simulink model "sistemaConControladorPID_R2022a"  (R2022a)
settings: Solver=VariableStepAuto  StartTime=0.0  StopTime=Ts  RelTol=1e-3
libraries: dspsrcs4 x1, slpidlib x1, cstblocks x1
settings Model: Creator=chris  LastModifiedBy=chris
settings ModelReferenceCC: EnableRefExpFcnMdlSchedulingChecks=off
settings RTWCC: Description=Generic Real-Time Target

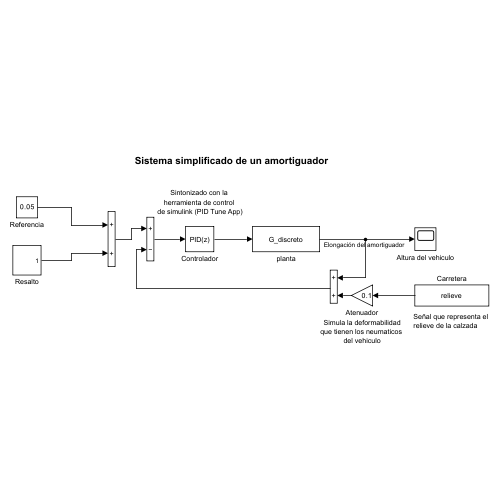
[thumbnail: Simulink's stored preview of the top-level diagram]
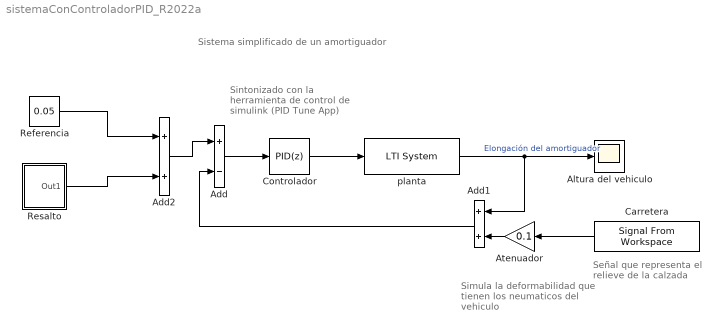
== system sistemaConControladorPID_R2022a ==
  note: Señal que representa el
      | relieve de la calzada
  note: Simula la deformabilidad
      | que tienen los neumaticos
      | del vehiculo
  note: Sistema simplificado de un amortiguador
  note: Sintonizado con la
      | herramienta de control
      | de simulink (PID Tune App)
  Add : Sum  Inputs=+-
  Add1 : Sum
  Add2 : Sum
  Altura del vehiculo : Scope
  Atenuador : Gain  Gain=0.1
  Carretera : dspsrcs4/Signal From Workspace  X=relieve  Ts=0.01  nsamps=1  OutputAfterFinalValue=Setting to zero  ignoreOrWarnInputAndFrameLengths=off  OutputFrames=off
  Controlador : slpidlib/PID Controller  Controller=PID  Form=Parallel  TimeDomain=Discrete-time  UseExternalTs=off  SampleTime=-1  IntegratorMethod=Forward Euler  FilterMethod=Forward Euler  ControllerParametersSource=internal  P=0.43918474089495  I=0.0612558030086578  UseKiTs=off  D=0.368923056503776  N=110.757221993081  UseFilter=on  TunerSelectOption=Transfer Function Based (PID Tuner App)  InitialConditionSource=internal  InitialConditionForIntegrator=0  InitialConditionForFilter=0  DifferentiatorICPrevScaledInput=0  ExternalReset=none  TrackingMode=off  Kt=1  LimitOutput=off  SatLimitsSource=internal  UpperSaturationLimit=inf  LowerSaturationLimit=-inf  LinearizeAsGain=off  AntiWindupMode=none  Kb=1  POutMin=[]  POutMax=[]  IOutMin=[]  IOutMax=[]  DOutMin=[]  DOutMax=[]  NOutMin=[]  NOutMax=[]  SumOutMin=[]  SumOutMax=[]  SaturationOutMin=[]  SaturationOutMax=[]  PParamMin=[]  PParamMax=[]  IParamMin=[]  IParamMax=[]  DParamMin=[]  DParamMax=[]  NParamMin=[]  NParamMax=[]  KbParamMin=[]  KbParamMax=[]  KtParamMin=[]  KtParamMax=[]  KbOutMin=[]  KbOutMax=[]  KtOutMin=[]  KtOutMax=[]  IntegratorOutMin=[]  IntegratorOutMax=[]  FilterOutMin=[]  FilterOutMax=[]  SumI1OutMin=[]  SumI1OutMax=[]  SumI2OutMin=[]  SumI2OutMax=[]  SumI3OutMin=[]  SumI3OutMax=[]  SumI4OutMin=[]  SumI4OutMax=[]  SumDOutMin=[]  SumDOutMax=[]  DifferentiatorOutMin=[]  DifferentiatorOutMax=[]  FilterDiffOutCoefMin=[]  FilterDiffOutCoefMax=[]  ReciprocalOutMin=[]  ReciprocalOutMax=[]  SumDenOutMin=[]  SumDenOutMax=[]  SumNumOutMin=[]  SumNumOutMax=[]  DivideOutMin=[]  DivideOutMax=[]  UdiffTsProdOutMin=[]  UdiffTsProdOutMax=[]  NTsProdOutMin=[]  NTsProdOutMax=[]  UintegralTsProdOutMin=[]  UintegralTsProdOutMax=[]  UngainTsProdOutMin=[]  UngainTsProdOutMax=[]  IntegratorContinuousStateAttributes=''  IntegratorStateMustResolveToSignalObject=off  IntegratorRTWStateStorageClass=Auto  FilterContinuousStateAttributes=''  FilterStateMustResolveToSignalObject=off  FilterRTWStateStorageClass=Auto  ParallelPVariant=InternalParameters  IdealPVariant=Disabled  IVariant=InternalParameters  DVariant=InternalParameters  IntegratorVariant=Discrete  SatVariant=Disabled  AWVariant=Passthrough  PCopyVariant=Disabled  TRVariant=Disabled  FdbkBlocksVariant=Forward  IdealPFdbkVariant=Disabled  SatFdbkVariant=Disabled  DerivativeFilterVariant=ForwardEulerFilter  NVariant=InternalParameters  NCopyVariant=Disabled  FilterICVariant=InternalICsFilter  IntegratorICVariant=InternalICs  ExternalResetVariant=Disabled  TRSumVariant=Passthrough  SumFdbkVariant=Disabled  SumVariant=Sum_PID  TsampFilterVariant=InternalTs  TsampNgainVariant=Passthrough  TsampIntegralVariant=Disabled_SignalSpec  ExternalSaturationOutDataTypeStr=Inherit: Same as second input
  Referencia : Constant  Value=0.05
  Resalto : Subsystem
  planta : cstblocks/LTI System  sys=G_discreto  IC=[]
  wires:
  Controlador/1 -> planta/1
  Add/1 -> Controlador/1
  planta/1 -> Add1/1, Altura del vehiculo/1  "Elongación del amortiguador"
  Add1/1 -> Add/2
  Atenuador/1 -> Add1/2
  Carretera/1 -> Atenuador/1
  Referencia/1 -> Add2/1
  Add2/1 -> Add/1
  Resalto/1(Out1) -> Add2/2

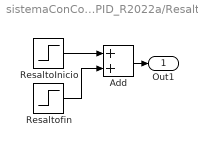
== system sistemaConControladorPID_R2022a/Resalto ==
  Add : Sum
  ResaltoInicio : Step  Time=4.5  After=0.12  SampleTime=0
  Resaltofin : Step  Time=10.5  After=-0.12  SampleTime=0
  Out1 : Outport
  wires:
  Resaltofin/1 -> Add/2
  Add/1 -> Out1/1
  ResaltoInicio/1 -> Add/1
